simulink model "SIL"  (R2025b)
settings: Solver=FixedStepDiscrete  StartTime=0.0  StopTime=inf  FixedStep=0.01  RelTol=1e-3
settings Model: NumberOfSteps=10  Creator=Gabriel  LastModifiedBy=Gabriel
settings SFSimCC: SimCustomInitializer=SS_App_Init();  SimUserIncludeDirs="\"C:\\Users\\Gabriel\\Desktop\\Pós graduação - Sistemas automotivos\\projeto_final\\coding_local\\include\""
settings SFSimCC: SimCustomHeaderCode=|
  | #include "ss_app.h"
  | 
  | #include "ss_input_proc.h"
  | 
  | #include "ss_operation.h"
  | 
  | #include "ss_types.h"
  | 
  | #include "ss_calib.h"
  | 
  | #include "ss_timer.h"
  | 
  | #include "ss_inhibit_safety_conditions.h"
settings SFSimCC: SimUserSources=|
  | "C:\Users\Gabriel\Desktop\Pós graduação - Sistemas automotivos\projeto_final\coding_local\src\ss_operation.c"
  | 
  | "C:\Users\Gabriel\Desktop\Pós graduação - Sistemas automotivos\projeto_final\coding_local\src\ss_input_proc.c"
  | 
  | "C:\Users\Gabriel\Desktop\Pós graduação - Sistemas automotivos\projeto_final\coding_local\src\ss_app.c"
  | 
  | "C:\Users\Gabriel\Desktop\Pós graduação - Sistemas automotivos\projeto_final\coding_local\src\timer.c"
  | 
  | "C:\Users\Gabriel\Desktop\Pós graduação - Sistemas automotivos\projeto_final\coding_local\src\ss_inhibit_safety_conditions.c"

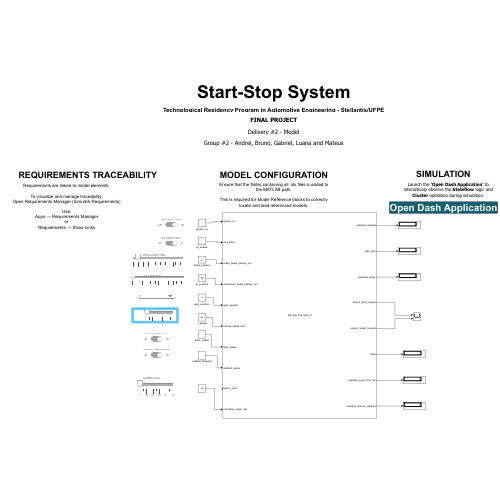
[thumbnail: Simulink's stored preview of the top-level diagram]
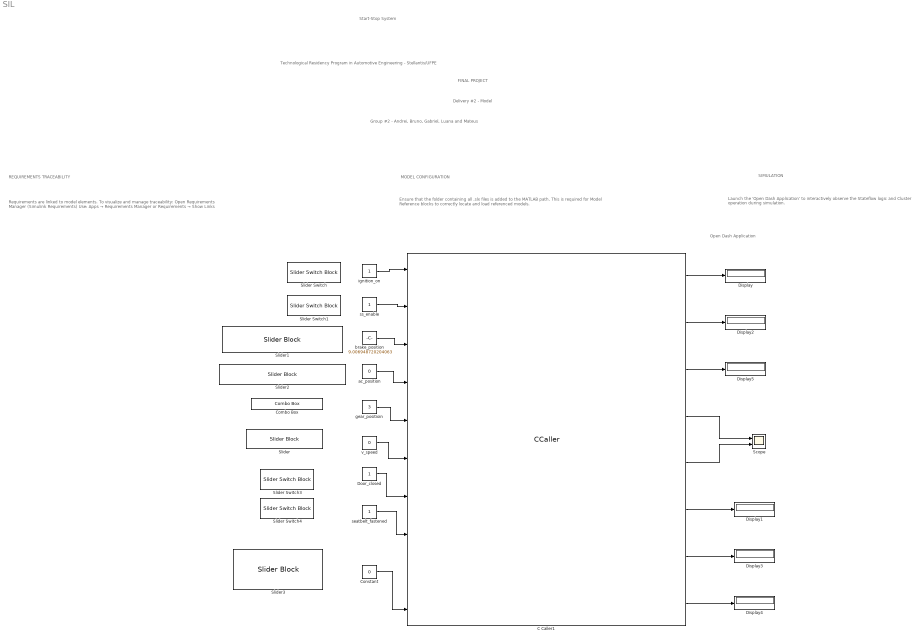
== system SIL ==
  note: Open Dash Application
  note: Technological Residency Program in Automotive Engineering - Stellantis/UFPE
  note: Start-Stop System
  note: FINAL PROJECT
  note: Group #2 - Andrei, Bruno, Gabriel, Luana and Mateus
  note: Delivery #2 - Model
  note: SIMULATION
  note: Launch the 'Open Dash Application' to interactively observe the Stateflow logic and Cluster operation during simulation.
  note: REQUIREMENTS TRACEABILITY
  note: Requirements are linked to model elements.
      |
      | To visualize and manage traceability:
      | Open Requirements Manager (Simulink Requirements)
      |
      | Use:
      | Apps → Requirements Manager
      | or
      | Requirements → Show Links
  note: Ensure that the folder containing all .slx files is added to the MATLAB path.
      |
      | This is required for Model Reference blocks to correctly locate and load referenced models.
  note: MODEL CONFIGURATION
  C Caller1 : CCaller  FunctionName=SS_App_Run10ms_If  PortSpecificationStruct="%)30     .    >\"    8    (     @         %    \"    !(    !     0         %  0 \"0    $    _    07)G3F%M90  4&]R=$YA;64 4V-O<&4     26YD97@     5'EP90      4VEZ90      27-';&]B86P   X   !     !@    @    $          4    (     0    L    !         !     +    :6=N:71I;VY?;VX       X   !     !@    @    $          4    (     0    L    !         !     +    :6=N:71I;VY?;VX       X    X    !@    @    $    ...(+10824 chars)"  SampleTime=0.01
  Combo Box : ComboBox  LabelPosition=Hide  SelectedLabel=D
  Constant : Constant  Value=0  OutDataTypeStr=single
  Display{,1..5} (6 alike) : Display
  Door_closed : Constant  OutDataTypeStr=boolean
  Scope : Scope  NumInputPorts=2
  Slider{,1..3} (4 alike) : SliderBlock
  Slider Switch{,1,3..4} (4 alike) : SliderSwitchBlock
  ac_position : Constant  Value=0  OutDataTypeStr=single
  brake_position : Constant  Value=9.006948720204063  OutDataTypeStr=single
  gear_positioin : Constant  Value=3  OutDataTypeStr=int32
  ignition_on : Constant  OutDataTypeStr=boolean
  seatbelt_fastened : Constant  OutDataTypeStr=boolean
  ss_enable : Constant  OutDataTypeStr=boolean
  v_speed : Constant  Value=0  OutDataTypeStr=single
  wires:
  ignition_on/1 -> C Caller1/1
  ss_enable/1 -> C Caller1/2
  brake_position/1 -> C Caller1/3
  ac_position/1 -> C Caller1/4
  gear_positioin/1 -> C Caller1/5
  Door_closed/1 -> C Caller1/7
  seatbelt_fastened/1 -> C Caller1/8
  Constant/1 -> C Caller1/10
  C Caller1/1 -> Display/1
  C Caller1/2 -> Display2/1
  C Caller1/4 -> Scope/1
  C Caller1/6 -> Display1/1
  v_speed/1 -> C Caller1/6
  C Caller1/3 -> Display5/1
  C Caller1/5 -> Scope/2
  C Caller1/7 -> Display3/1
  C Caller1/8 -> Display4/1
